simulink subsystem "EKF"  (R2024a)
settings: Solver=VariableStepAuto  StartTime=0.0  StopTime=10.0  RelTol=1e-3
undefined symbols (not defined in the file): N_KF, P0, Q_KF, R_KF, x0
settings Model: Creator=Bocchio  LastModifiedBy=Bocchio

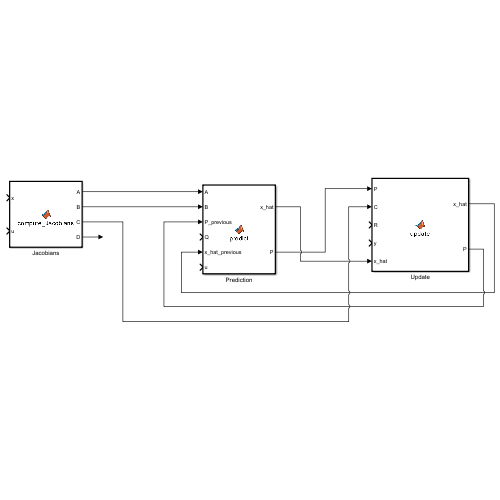
[thumbnail: Simulink's stored preview of the top-level diagram]
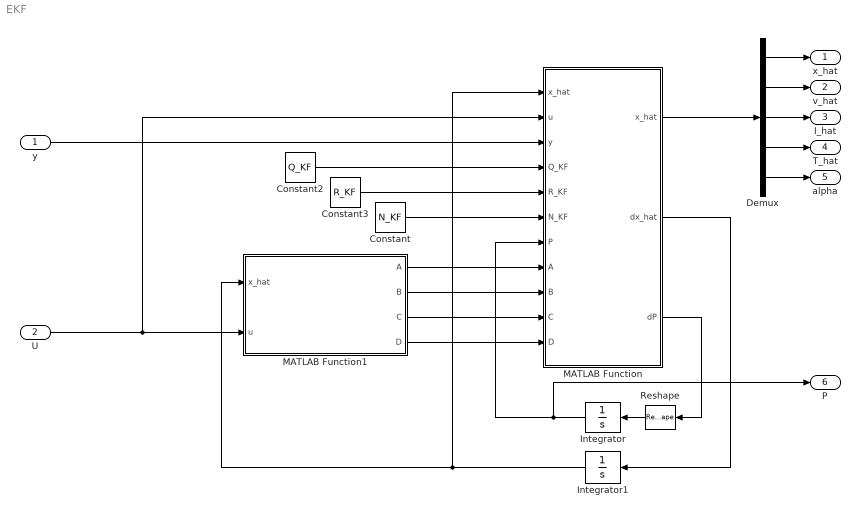
== system EKF ==
  y : Inport
  U : Inport  Port=2
  Constant : Constant  Value=N_KF
  Constant2 : Constant  Value=Q_KF
  Constant3 : Constant  Value=R_KF
  Demux : Demux  Outputs=5
  Integrator : Integrator  InitialCondition=P0(:)
  Integrator1 : Integrator  InitialCondition=x0
  MATLAB Function : MATLAB Function  TreatAsAtomicUnit=on
  MATLAB Function1 : MATLAB Function  TreatAsAtomicUnit=on
  Reshape : Reshape
  x_hat : Outport
  v_hat : Outport  Port=2
  I_hat : Outport  Port=3
  T_hat : Outport  Port=4
  alpha : Outport  Port=5
  P : Outport  Port=6
  wires:
  MATLAB Function1/3(C) -> MATLAB Function/10(C)
  MATLAB Function1/2(B) -> MATLAB Function/9(B)
  Constant2/1 -> MATLAB Function/4(Q_KF)
  MATLAB Function1/1(A) -> MATLAB Function/8(A)
  MATLAB Function/2(dx_hat) -> Integrator1/1
  Demux/3 -> I_hat/1
  y/1 -> MATLAB Function/3(y)
  MATLAB Function1/4(D) -> MATLAB Function/11(D)
  Constant3/1 -> MATLAB Function/5(R_KF)
  Constant/1 -> MATLAB Function/6(N_KF)
  MATLAB Function/1(x_hat) -> Demux/1
  MATLAB Function/3(dP) -> Reshape/1
  Integrator1/1 -> MATLAB Function1/1(x_hat), MATLAB Function/1("x_hat ")
  U/1 -> MATLAB Function/2(u), MATLAB Function1/2(u)
  Demux/1 -> x_hat/1
  Demux/2 -> v_hat/1
  Demux/5 -> alpha/1
  Integrator/1 -> MATLAB Function/7(P), P/1
  Reshape/1 -> Integrator/1
  Demux/4 -> T_hat/1

== matlab function EKF/MATLAB Function ==
  data: x_hat output; x_hat input; u input; dx_hat output; y input; dP output; Q_KF input; R_KF input; N_KF input; P input; A input; B input; C input; D input
function [x_hat, dx_hat, dP]  = EKF(x_hat, u, y, Q_KF, R_KF, N_KF, P, A, B, C, D)

% ARE
P = reshape(P, size(A));
dP = (A*P + P*A' + Q_KF - P*C'* R_KF^-1 *C*P);

% Optimal gain
K = (P*C') / R_KF;

dx_hat = A(:, 1:end-1)*x_hat(1:end-1) + B*u + K*(y - C*x_hat);

end

== matlab function EKF/MATLAB Function1 ==
  settings: updateMethod=DISCRETE
  data: A output; B output; C output; D output; x_hat input; u input
function [A, B, C, D] = ABCD_lagrangian_1DOF(x_hat, u)

%% Parameters
C_T = 449; %[J/(kg*°k)] Thermal capacity
h = 80e+3; %[W/k] Thermal dissipation coefficient
T_env = 22; %[] Ambient temperature
m = 0.5; %[kg] Mass of the piston
L0 = 1e-1; %[H] Inductance at a reference temperature
beta1 = 1e-5; %[H/°C] Coefficients for the T-dependent inductance
beta2 = 1e-7; %[H/°C^2] Coefficients for the T-dependent inductance

c = 1e-2; %[] Damping
k1 = 10; %[N/m] Coefficients for the x-dependent stiffness
k3 = 2; %[N/m^3] Coefficients for the x-dependent stiffness

% alpha0 = 1.2; %[N/A] Force constant

R = 5; %[ohm] Resistance

%% ABCD for Extended Kalman filter + parameter identification

L = @(T) L0 + beta1 * T + beta2 * T^2;
dLdT = @(T) beta1 + 2*beta2 * T;
ddLddT = @(T) 2*beta2; %#ok<NASGU>


% A coefficients
a11 = 0;
a12 = 1;
a13 = 0;
a14 = 0;

a21 = 1 / m * (-k1 -3*k3*x_hat(1)^2);
a22 = 1 / m * (-c);
a23 = 1 / m * (x_hat(5));
a24 = 0;

a31 = 0;
a32 = 0;
a33 = -R / L(x_hat(4));
a34 = (-R*x_hat(3) + u) * ( -1 / L(x_hat(4))^2 ) * dLdT(x_hat(4));

a41 = 0;
a42 = 0;
a43 = 1 / C_T * (2*R*x_hat(3));
a44 = 1 / C_T * (-h);

% B coefficients
b1 = 0;
b2 = 0;
b3 = 1 / L(x_hat(4));
b4 = 0;

% C coefficients
c1 = 1;
c2 = 0;
c3 = 0;
c4 = 0;

% D coefficients
d1 = 0;


% State matrices
A = [
    a11 a12 a13 a14 0;
    a21 a22 a23 a24 1/m * x_hat(3);
    a31 a32 a33 a34 0;
    a41 a42 a43 a44 0;
      0   0   0   0 0
    ];

B = [
    b1;
    b2;
    b3;
    b4;
     0
    ];

C = [c1 c2 c3 c4 0];

D = [d1 0];

end
